simulink model "mpu6050"  (R2017b)
settings: Solver=FixedStepDiscrete  StartTime=0.0  StopTime=0.5  FixedStep=0.01  RelTol=1e-3
undefined symbols (not defined in the file): DiscIntNeverNeededParam, KiRollAttitude, KpRollAttitude, mpu6050
libraries: simulink x6, GPIO_Lib x3, TIMERS_Lib x2, STM32_Config_Lib x1
(part 1 of 2)
settings Model: Creator=edupc  LastModifiedBy=edupc
settings OptimizationCC: DefaultParameterBehavior=Inlined  PassReuseOutputArgsAs=Individual arguments
settings DebuggingCC: ParameterTunabilityLossMsg=error
settings HardwareCC: ProdBitPerPointer=32  ProdBitPerSizeT=32  ProdBitPerPtrDiffT=32  ProdLargestAtomicInteger=Integer  ProdWordSize=32  ProdHWDeviceType=STMicroelectronics->STM32 32-bit Cortex-M
settings SFSimCC: SimCustomHeaderCode="#include \"mac.h\""  SimUserSources=mac.c  MATLABDynamicMemAlloc=off
settings RTWCC: SystemTargetFile=stm32.tlc  TemplateMakefile=stm32.tmf  Description=stm32 (Embedded Target)  GenerateReport=on  IncludeHyperlinkInReport=on  GenerateTraceInfo=on  GenerateTraceReport=on  GenerateTraceReportSl=on  GenerateTraceReportSf=on  GenerateTraceReportEml=on
settings RTWCC: CustomHeaderCode=|
  | #include "printfFile.h"
  | #include "global.h"
settings CodeAppCC: ForceParamTrailComments=on  IgnoreCustomStorageClasses=off  MaxIdLength=64  OperatorAnnotations=on  SimulinkDataObjDesc=on  SFDataObjDesc=on  CustomSymbolStrType=$N$R$M  SimulinkBlockComments=off
settings STFCustomTargetCC: CodeReplacementLibrary=ARM CMSIS SIN COS  MultiwordLength=256  ParMdlRefBuildCompliant=on  IncludeMdlTerminateFcn=off  CombineOutputUpdateFcns=on  ERTCustomFileBanners=on  SupportContinuousTime=off  SupportNonInlinedSFcns=off  RemoveResetFunc=on  MATLABClassNameForMDSCustomization=Simulink.SoftwareTarget.ERTCustomization  GRTInterface=off  SystemTargetFile=stm32.tlc
settings ERTTargetCC: CodeReplacementLibrary=ARM CMSIS SIN COS  CompOptLevelCompliant=off  ConcurrentExecutionCompliant=off  IncludeMdlTerminateFcn=off  ModelStepFunctionPrototypeControlCompliant=off  CPPClassGenCompliant=off  UseToolchainInfoCompliant=off  ExtModeStaticAllocSize=256  ExtModeMexArgs=0,1,115200,10  InlinedParameterPlacement=NonHierarchical  ERTSrcFileBannerTemplate=sourceFileTemplate.cgt  ERTHdrFileBannerTemplate=sourceFileTemplate.cgt  ERTDataSrcFileTemplate=sourceFileTemplate.cgt  ERTDataHdrFileTemplate=sourceFileTemplate.cgt  ERTCustomFileTemplate=customRoutineProcess.tlc

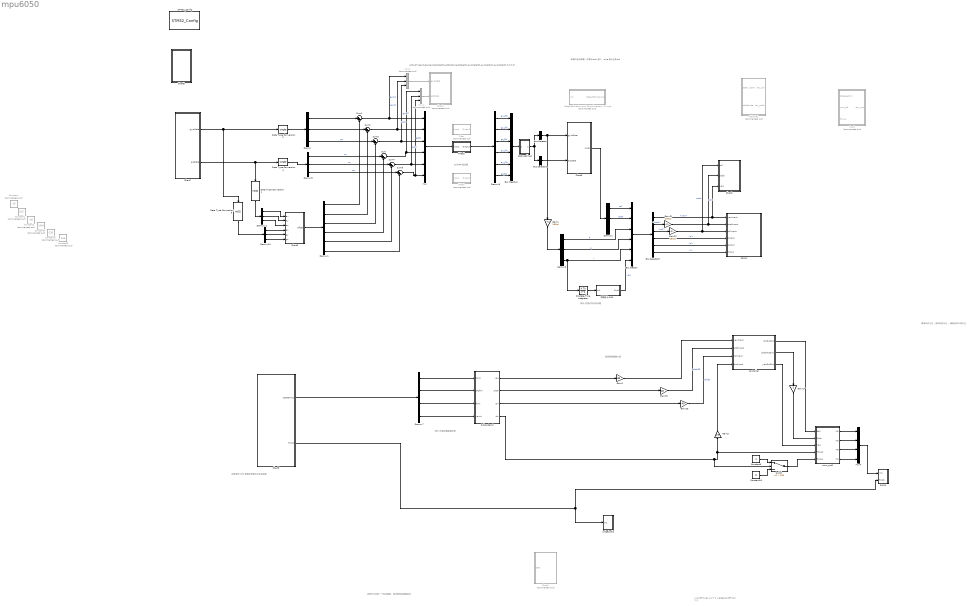
== system mpu6050 ==
  note: //				printf("over run");
      | 			}
      | //      else{printf("no\r\n");}
  note: 50Hz的遥控器数据处理
  note: 角速度期望最大值
  note: 10阶FIR滤波器
  note: ANO_DT_Send_Senser(accData[0],accData[1],accData[2],gyroData[0],gyroData[1],gyroData[2],0,0,0,0);
  note: 这里可以先放一个发送函数，测试是否有数据丢失
  note: 这里添加了PID参数回传确认的发送函数
  note: 航向 这里还存在些问题
  note: 横滚向右为正，俯仰向前为正，
      | 偏航逆时针转为正
  note: 移植的姿态解算，陀螺仪rad/s输入，ouler输出也是rad
  Attitude1 : Subsystem  Commented=on  TreatAsAtomicUnit=on
  Bus Creator : BusCreator  Inputs=6
  Bus Creator4 : BusCreator  Inputs=6
  Bus Selector : BusSelector  OutputSignals=p,q,r  OutputAsBus=on
  Bus Selector1 : BusSelector  OutputSignals=x_acc,y_acc,z_acc  OutputAsBus=on
  Bus Selector3 : BusSelector  OutputSignals=yaw,pitch,roll,p,q,r
  Chart1 : Stateflow chart  TreatAsAtomicUnit=on
  Chart2 : Stateflow chart  Commented=on  TreatAsAtomicUnit=on
  Chart3 : Stateflow chart  TreatAsAtomicUnit=on
  Chart4 : Stateflow chart  Commented=on  TreatAsAtomicUnit=on
  Chart5 : Stateflow chart  TreatAsAtomicUnit=on
  Chart6 : Stateflow chart  TreatAsAtomicUnit=on
  Chart7 : Stateflow chart  TreatAsAtomicUnit=on
  Chart8 : Stateflow chart  Priority=1  TreatAsAtomicUnit=on
  Constant : Constant  Commented=on  Value=-29  OutDataTypeStr=single
  Constant1 : Constant  Commented=on  Value=16.5  OutDataTypeStr=single
  Constant10 : Constant  Value=0  OutDataTypeStr=single
  Constant2 : Constant  Commented=on  Value=-36  OutDataTypeStr=single
  Constant3 : Constant  Commented=on  Value=1040  OutDataTypeStr=single
  Constant4 : Constant  Commented=on  Value=-130  OutDataTypeStr=single
  Constant5 : Constant  Commented=on  Value=516  OutDataTypeStr=single
  Constant9 : Constant  OutDataTypeStr=single
  Data Type Conversion1 : DataTypeConversion  OutDataTypeStr=int32
  Data Type Conversion2 : DataTypeConversion  OutDataTypeStr=single  RndMeth=Nearest
  Data Type Conversion4 : DataTypeConversion  OutDataTypeStr=single  RndMeth=Nearest
  Data Type Conversion5 : DataTypeConversion  OutDataTypeStr=int32
  Demux{,2..3,9..11} (6 alike) : Demux  Outputs=3
  Demux1 : Demux  Outputs=6
  Demux7 : Demux
  Demux8 : Demux  Outputs=6
  Discrete-Time Integrator : DiscreteIntegrator  gainval=1  InitialConditionSetting=State (most efficient)  SampleTime=-1  ICPrevOutput=DiscIntNeverNeededParam  ICPrevScaledInput=DiscIntNeverNeededParam
  Filter : Subsystem  Tag=FilterWizardSubSystem  Commented=on
      settings: ErrorFcn=dspFilterRealizedInBasicElemsAlgLoopErrFcnCallback
  Filter1 : Subsystem  Tag=FilterWizardSubSystem  Commented=on
      settings: ErrorFcn=dspFilterRealizedInBasicElemsAlgLoopErrFcnCallback
  Filter2 : Subsystem  Tag=FilterWizardSubSystem
      settings: ErrorFcn=dspFilterRealizedInBasicElemsAlgLoopErrFcnCallback
  Gain1 : Gain  Gain=180/pi
  Gain17 : Gain  Gain=-1  ParamDataTypeStr=single  OutDataTypeStr=single
  Gain19 : Gain  Gain=40  ParamDataTypeStr=single
  Gain2 : Gain  Gain=180  ParamDataTypeStr=single
  Gain20 : Gain  Gain=40
  Gain21 : Gain  Gain=180/pi
  Gain22 : Gain  Gain=180/pi
  Gain3 : Gain  Gain=0.5  ParamDataTypeStr=single
  Mux : Mux  Inputs=6
  Mux1 : Mux  Commented=on  Inputs=3
  Mux2 : Mux  Commented=on  Inputs=3
  Mux4 : Mux
  PWM1 : Subsystem  TreatAsAtomicUnit=on
  STM32_Config : STM32_Config_Lib/STM32_Config  Priority=0  Project_Path=.\mpu6050\  Config_File=mpu6050.ioc  MCU_Name=STM32F103T8Ux
      settings: SourceProductName=Target Support Package - STM32 Adapter
  State Estimation and Complimentary Mixing1 : Subsystem  Commented=on  mask{EAComp=0.95}
      mask prompts: EAComp "Complimentary Filter Alpha:"
      mask TypeOptions EAComp: Complimentary Filter/EAComp
  Subsystem2 : Subsystem  TreatAsAtomicUnit=on
  Sum{,1..5} (6 alike) : Sum  Inputs=|+-
  Switch : Switch  Criteria=u2 > Threshold  Threshold=100
  Yaw1 : Subsystem  Commented=on  TreatAsAtomicUnit=on
  controller : Stateflow chart  TreatAsAtomicUnit=on
  data scaling1 : Subsystem
  judgeLock2 : Subsystem  TreatAsAtomicUnit=on
  pwm_out2 : MATLAB Function  TreatAsAtomicUnit=on
  sensor : Stateflow chart  TreatAsAtomicUnit=on
  限幅到+-180， : Subsystem
  wires:
  Data Type Conversion1/1 -> Demux11/1
  Demux10/1 -> Chart6/4(gx)
  Demux1/6 -> Sum5/2
  Demux11/1 -> Chart6/1(ax)
  Demux1/4 -> Sum/2
  Demux10/2 -> Chart6/5(gy)
  Chart7/2(accData) -> Data Type Conversion1/1, Data Type Conversion4/1
  Sum/1 -> Mux1/1, Mux/4  "accX"
  Demux1/2 -> Sum2/2
  Demux/2 -> Sum2/1
  Data Type Conversion2/1 -> Demux/1
  Sum1/1 -> Mux2/1, Mux/1  "gyroX"
  Sum4/1 -> Mux1/2, Mux/5  "accY"
  Demux9/3 -> Sum5/1  "az"
  Demux11/2 -> Chart6/2(ay)
  Demux9/2 -> Sum4/1  "ay"
  Demux11/3 -> Chart6/3(az)
  Sum5/1 -> Mux1/3, Mux/6  "accZ"
  Demux9/1 -> Sum/1  "ax"
  Demux10/3 -> Chart6/6(gz)
  Chart7/1(gyroData) -> Data Type Conversion2/1, Data Type Conversion5/1
  Demux1/1 -> Sum1/2
  Sum3/1 -> Mux2/3, Mux/3  "gyroZ"
  Demux/3 -> Sum3/1  "gz"
  Demux/1 -> Sum1/1
  Data Type Conversion5/1 -> Demux10/1
  Data Type Conversion4/1 -> Demux9/1
  Demux1/5 -> Sum4/2
  Demux1/3 -> Sum3/2
  Sum2/1 -> Mux2/2, Mux/2  "gryoY"
  Demux8/5 -> Bus Creator4/5  "ay_filt"
  Demux8/1 -> Bus Creator4/1  "gx_filt"
  Mux/1 -> Filter2/1(Input)
  Demux8/2 -> Bus Creator4/2  "gy_filt"
  Demux8/3 -> Bus Creator4/3  "gz_filt"
  Demux8/4 -> Bus Creator4/4  "ax_filt"
  Bus Creator4/1 -> data scaling1/1(In1)
  Demux8/6 -> Bus Creator4/6  "az_filt"
  Chart5/1(rcDataTmp) -> Demux7/1
  controller/2(pitchOutSim) -> Gain17/1
  Mux4/1 -> PWM1/1(In1)
  Subsystem2/3(roll) -> Gain20/1
  pwm_out2/2(M2) -> Mux4/2
  Chart5/2(FlyOk) -> PWM1/2(flyOk), judgeLock2/1(In1)
  Demux7/4 -> Subsystem2/4(yawIn)
  Subsystem2/2(pitch) -> Gain19/1
  Subsystem2/1(yaw) -> Gain2/1
  pwm_out2/1(M1) -> Mux4/1
  pwm_out2/4(M4) -> Mux4/4
  pwm_out2/3(M3) -> Mux4/3
  Demux7/2 -> Subsystem2/2(pitchIn)
  Subsystem2/4(thr) -> Switch/2, pwm_out2/4(Thrust), Gain3/1
  Demux7/3 -> Subsystem2/3(thrIn)
  Demux7/1 -> Subsystem2/1(rollIn)
  Chart3/1(ouler) -> Demux2/1
  data scaling1/1(Out1) -> Bus Selector1/1, Bus Selector/1
  Bus Selector1/1 -> Chart3/2(accData)
  Bus Selector/1 -> Chart3/1(gyroData), Gain1/1
  Demux2/1 -> Bus Creator/1  "roll"
  Demux2/2 -> Bus Creator/2  "pitch"
  Bus Creator/1 -> Bus Selector3/1
  Demux3/1 -> Bus Creator/3  "p"
  Demux3/2 -> Bus Creator/4  "q"
  Demux3/3 -> Discrete-Time Integrator/1, Bus Creator/5  "r"
  Filter2/1(Output) -> Demux8/1
  Discrete-Time Integrator/1 -> 限幅到+-180，/1(In1)
  限幅到+-180，/1(Out1) -> Bus Creator/6  "yaw"
  Gain17/1 -> pwm_out2/2(Pitch)
  Chart6/1(offset) -> Demux1/1
  Mux1/1 -> Chart4/2(accData)
  Mux2/1 -> Chart4/1(gyroData)
  Gain2/1 -> controller/1(yawInput)
  Gain3/1 -> controller/4(throInput)
  Constant10/1 -> Switch/3
  Constant9/1 -> Switch/1
  Switch/1 -> pwm_out2/5(thrLow)
  Gain19/1 -> controller/2(pitchInput)  "pitchCtl"
  Gain20/1 -> controller/3(rollInput)  "rollCtl"
  Bus Selector3/1 -> Chart1/3(yaw), sensor/1(yawInput)  "<yaw>"
  Bus Selector3/2 -> Gain21/1  "<pitch>"
  Bus Selector3/3 -> Gain22/1  "<roll>"
  Gain21/1 -> Chart1/2(pitch), sensor/2(pitchInput)  "roll"
  Gain22/1 -> Chart1/1(roll), sensor/3(rollInput)  "pitch"
  Bus Selector3/4 -> sensor/4(pInput)  "<p>"
  Bus Selector3/5 -> sensor/5(qInput)  "<q>"
  Bus Selector3/6 -> sensor/6(rInput)  "<r>"
  controller/3(yawOutSim) -> pwm_out2/3(Yaw)
  Gain1/1 -> Demux3/1
  controller/1(rollOutSim) -> pwm_out2/1(Roll)

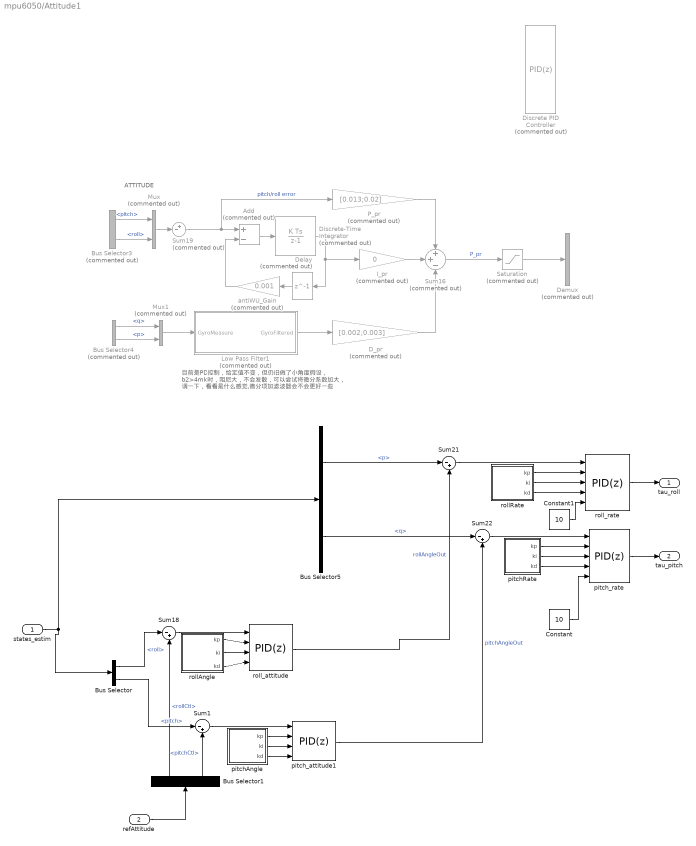
== system mpu6050/Attitude1 ==
  note: 目前是PD控制，给定值不变，但仍旧做了小角度假设，
      | b2>4mk时，阻尼大，不会发散，可以尝试将微分系数加大，
      | 调一下，看看是什么感觉,微分项加滤波器会不会更好一些
  note: ATTITUDE
  states_estim : Inport
  refAttitude : Inport  Port=2
  Add : Sum  Commented=on  Inputs=+-
  Bus Selector : BusSelector  OutputSignals=roll,pitch
  Bus Selector1 : BusSelector  OutputSignals=rollCtl,pitchCtl
  Bus Selector3 : BusSelector  Commented=on  OutputSignals=pitch,roll
  Bus Selector4 : BusSelector  Commented=on  OutputSignals=q,p
  Bus Selector5 : BusSelector  OutputSignals=p,q
  Constant : Constant  Value=10  OutDataTypeStr=int8
  Constant1 : Constant  Value=10  OutDataTypeStr=int8
  D_pr : Gain  Commented=on  Gain=[0.002;0.003]  ParamDataTypeStr=single  OutDataTypeStr=single
  Delay : Delay  Commented=on  DelayLength=1  InitialCondition=0
  Demux : Demux  Commented=on  Outputs=2
  Discrete PID Controller : simulink/Continuous/PID Controller  Commented=on  Controller=PID  TimeDomain=Discrete-time  SampleTime=-1  IntegratorMethod=Backward Euler  FilterMethod=Backward Euler  Form=Parallel  UseFilter=on  ControllerParametersSource=external  P=1  I=1  D=0  N=100  InitialConditionSource=internal  InitialConditionForIntegrator=0  InitialConditionForFilter=0  ExternalReset=none  LimitOutput=off  UpperSaturationLimit=inf  LowerSaturationLimit=-inf  LinearizeAsGain=off  AntiWindupMode=none  Kb=1  TrackingMode=off  Kt=1  PParamMin=[]  PParamMax=[]  IParamMin=[]  IParamMax=[]  DParamMin=[]  DParamMax=[]  NParamMin=[]  NParamMax=[]  KbParamMin=[]  KbParamMax=[]  KtParamMin=[]  KtParamMax=[]  POutMin=[]  POutMax=[]  IOutMin=[]  IOutMax=[]  DOutMin=[]  DOutMax=[]  NOutMin=[]  NOutMax=[]  KbOutMin=[]  KbOutMax=[]  KtOutMin=[]  KtOutMax=[]  IntegratorOutMin=[]  IntegratorOutMax=[]  FilterOutMin=[]  FilterOutMax=[]  SumOutMin=[]  SumOutMax=[]  SumI1OutMin=[]  SumI1OutMax=[]  SumI2OutMin=[]  SumI2OutMax=[]  SumI3OutMin=[]  SumI3OutMax=[]  SumDOutMin=[]  SumDOutMax=[]  SaturationOutMin=[]  SaturationOutMax=[]  IntegratorContinuousStateAttributes=''  IntegratorStateMustResolveToSignalObject=off  IntegratorRTWStateStorageClass=Auto  FilterContinuousStateAttributes=''  FilterStateMustResolveToSignalObject=off  FilterRTWStateStorageClass=Auto  DifferentiatorICPrevScaledInput=0  DifferentiatorOutMin=[]  DifferentiatorOutMax=[]  InitialConditionSetting=State (most efficient)  FilterDiffOutCoefMin=[]  FilterDiffOutCoefMax=[]  SumDenOutMin=[]  SumDenOutMax=[]  SumNumOutMin=[]  SumNumOutMax=[]  ReciprocalOutMin=[]  ReciprocalOutMax=[]  DivideOutMin=[]  DivideOutMax=[]  TunerSelectOption=Transfer Function Based (PID Tuner App)
  Discrete-Time Integrator : DiscreteIntegrator  Commented=on  InitialConditionSetting=State (most efficient)  SampleTime=-1  LimitOutput=on  UpperSaturationLimit=0.1  LowerSaturationLimit=-0.1  ICPrevOutput=DiscIntNeverNeededParam  ICPrevScaledInput=DiscIntNeverNeededParam
  I_pr : Gain  Commented=on  Gain=0  ParamDataTypeStr=single  OutDataTypeStr=single
  Low Pass Filter1 : Subsystem  Commented=on
  Mux : Mux  Commented=on  Inputs=2
  Mux1 : Mux  Commented=on  Inputs=2
  P_pr : Gain  Commented=on  Gain=[0.013;0.02]  ParamDataTypeStr=single  OutDataTypeStr=single
  Saturation : Saturate  Commented=on  UpperLimit=0.2  LowerLimit=-0.2
  Sum{1,18,21..22} (4 alike) : Sum  Inputs=|-+
  Sum16 : Sum  Commented=on  Inputs=++-  AccumDataTypeStr=single  OutDataTypeStr=single  SaturateOnIntegerOverflow=on
  Sum19 : Sum  Commented=on  Inputs=+-|
  antiWU_Gain : Gain  Commented=on  Gain=0.001
  pitchAngle : Stateflow chart  TreatAsAtomicUnit=on
  pitchRate : Stateflow chart  TreatAsAtomicUnit=on
  pitch_attitude1 : simulink/Continuous/PID Controller  Controller=PID  TimeDomain=Discrete-time  SampleTime=-1  IntegratorMethod=Forward Euler  FilterMethod=Forward Euler  Form=Parallel  UseFilter=off  ControllerParametersSource=external  P=KpRollAttitude  I=KiRollAttitude  D=0.01  N=100  InitialConditionSource=internal  InitialConditionForIntegrator=0  InitialConditionForFilter=0  ExternalReset=none  LimitOutput=on  UpperSaturationLimit=300  LowerSaturationLimit=-300  LinearizeAsGain=on  AntiWindupMode=back-calculation  Kb=2  TrackingMode=off  Kt=1  PParamMin=[]  PParamMax=[]  IParamMin=[]  IParamMax=[]  DParamMin=[]  DParamMax=[]  NParamMin=[]  NParamMax=[]  KbParamMin=[]  KbParamMax=[]  KtParamMin=[]  KtParamMax=[]  POutMin=[]  POutMax=[]  IOutMin=[-10]  IOutMax=[10]  DOutMin=[]  DOutMax=[]  NOutMin=[]  NOutMax=[]  KbOutMin=[]  KbOutMax=[]  KtOutMin=[]  KtOutMax=[]  IntegratorOutMin=[]  IntegratorOutMax=[]  FilterOutMin=[]  FilterOutMax=[]  SumOutMin=[]  SumOutMax=[]  SumI1OutMin=[]  SumI1OutMax=[]  SumI2OutMin=[]  SumI2OutMax=[]  SumI3OutMin=[]  SumI3OutMax=[]  SumDOutMin=[]  SumDOutMax=[]  SaturationOutMin=[]  SaturationOutMax=[]  IntegratorContinuousStateAttributes=''  IntegratorStateMustResolveToSignalObject=off  IntegratorRTWStateStorageClass=Auto  FilterContinuousStateAttributes=''  FilterStateMustResolveToSignalObject=off  FilterRTWStateStorageClass=Auto  DifferentiatorICPrevScaledInput=0  DifferentiatorOutMin=[]  DifferentiatorOutMax=[]  InitialConditionSetting=State (most efficient)  FilterDiffOutCoefMin=[]  FilterDiffOutCoefMax=[]  SumDenOutMin=[]  SumDenOutMax=[]  SumNumOutMin=[]  SumNumOutMax=[]  ReciprocalOutMin=[]  ReciprocalOutMax=[]  DivideOutMin=[]  DivideOutMax=[]  TunerSelectOption=Transfer Function Based (PID Tuner App)
  pitch_rate : simulink/Continuous/PID Controller  Controller=PID  TimeDomain=Discrete-time  SampleTime=-1  IntegratorMethod=Forward Euler  FilterMethod=Forward Euler  Form=Parallel  UseFilter=on  ControllerParametersSource=external  P=KpRollAttitude  I=KiRollAttitude  D=0.01  N=100  InitialConditionSource=internal  InitialConditionForIntegrator=0  InitialConditionForFilter=0  ExternalReset=none  LimitOutput=on  UpperSaturationLimit=300  LowerSaturationLimit=-300  LinearizeAsGain=on  AntiWindupMode=clamping  Kb=2  TrackingMode=off  Kt=1  PParamMin=[]  PParamMax=[]  IParamMin=[]  IParamMax=[]  DParamMin=[]  DParamMax=[]  NParamMin=[]  NParamMax=[]  KbParamMin=[]  KbParamMax=[]  KtParamMin=[]  KtParamMax=[]  POutMin=[]  POutMax=[]  IOutMin=[]  IOutMax=[]  DOutMin=[]  DOutMax=[]  NOutMin=[]  NOutMax=[]  KbOutMin=[]  KbOutMax=[]  KtOutMin=[]  KtOutMax=[]  IntegratorOutMin=[-100]  IntegratorOutMax=[100]  FilterOutMin=[]  FilterOutMax=[]  SumOutMin=[]  SumOutMax=[]  SumI1OutMin=[]  SumI1OutMax=[]  SumI2OutMin=[]  SumI2OutMax=[]  SumI3OutMin=[]  SumI3OutMax=[]  SumDOutMin=[]  SumDOutMax=[]  SaturationOutMin=[]  SaturationOutMax=[]  IntegratorContinuousStateAttributes=''  IntegratorStateMustResolveToSignalObject=off  IntegratorRTWStateStorageClass=Auto  FilterContinuousStateAttributes=''  FilterStateMustResolveToSignalObject=off  FilterRTWStateStorageClass=Auto  DifferentiatorICPrevScaledInput=0  DifferentiatorOutMin=[]  DifferentiatorOutMax=[]  InitialConditionSetting=State (most efficient)  FilterDiffOutCoefMin=[]  FilterDiffOutCoefMax=[]  SumDenOutMin=[]  SumDenOutMax=[]  SumNumOutMin=[]  SumNumOutMax=[]  ReciprocalOutMin=[]  ReciprocalOutMax=[]  DivideOutMin=[]  DivideOutMax=[]  TunerSelectOption=Transfer Function Based (PID Tuner App)
  rollAngle : Stateflow chart  TreatAsAtomicUnit=on
  rollRate : Stateflow chart  TreatAsAtomicUnit=on
  roll_attitude : simulink/Continuous/PID Controller  Controller=PID  TimeDomain=Discrete-time  SampleTime=-1  IntegratorMethod=Forward Euler  FilterMethod=Forward Euler  Form=Parallel  UseFilter=off  ControllerParametersSource=external  P=KpRollAttitude  I=KiRollAttitude  D=0.01  N=100  InitialConditionSource=internal  InitialConditionForIntegrator=0  InitialConditionForFilter=0  ExternalReset=none  LimitOutput=on  UpperSaturationLimit=300  LowerSaturationLimit=-300  LinearizeAsGain=on  AntiWindupMode=back-calculation  Kb=2  TrackingMode=off  Kt=1  PParamMin=[]  PParamMax=[]  IParamMin=[]  IParamMax=[]  DParamMin=[]  DParamMax=[]  NParamMin=[]  NParamMax=[]  KbParamMin=[]  KbParamMax=[]  KtParamMin=[]  KtParamMax=[]  POutMin=[]  POutMax=[]  IOutMin=[-10]  IOutMax=[10]  DOutMin=[]  DOutMax=[]  NOutMin=[]  NOutMax=[]  KbOutMin=[]  KbOutMax=[]  KtOutMin=[]  KtOutMax=[]  IntegratorOutMin=[]  IntegratorOutMax=[]  FilterOutMin=[]  FilterOutMax=[]  SumOutMin=[]  SumOutMax=[]  SumI1OutMin=[]  SumI1OutMax=[]  SumI2OutMin=[]  SumI2OutMax=[]  SumI3OutMin=[]  SumI3OutMax=[]  SumDOutMin=[]  SumDOutMax=[]  SaturationOutMin=[]  SaturationOutMax=[]  IntegratorContinuousStateAttributes=''  IntegratorStateMustResolveToSignalObject=off  IntegratorRTWStateStorageClass=Auto  FilterContinuousStateAttributes=''  FilterStateMustResolveToSignalObject=off  FilterRTWStateStorageClass=Auto  DifferentiatorICPrevScaledInput=0  DifferentiatorOutMin=[]  DifferentiatorOutMax=[]  InitialConditionSetting=State (most efficient)  FilterDiffOutCoefMin=[]  FilterDiffOutCoefMax=[]  SumDenOutMin=[]  SumDenOutMax=[]  SumNumOutMin=[]  SumNumOutMax=[]  ReciprocalOutMin=[]  ReciprocalOutMax=[]  DivideOutMin=[]  DivideOutMax=[]  TunerSelectOption=Transfer Function Based (PID Tuner App)
  roll_rate : simulink/Continuous/PID Controller  Controller=PID  TimeDomain=Discrete-time  SampleTime=-1  IntegratorMethod=Forward Euler  FilterMethod=Forward Euler  Form=Parallel  UseFilter=on  ControllerParametersSource=external  P=KpRollAttitude  I=KiRollAttitude  D=0.01  N=100  InitialConditionSource=internal  InitialConditionForIntegrator=0  InitialConditionForFilter=0  ExternalReset=none  LimitOutput=on  UpperSaturationLimit=300  LowerSaturationLimit=-300  LinearizeAsGain=on  AntiWindupMode=clamping  Kb=2  TrackingMode=off  Kt=1  PParamMin=[]  PParamMax=[]  IParamMin=[]  IParamMax=[]  DParamMin=[]  DParamMax=[]  NParamMin=[]  NParamMax=[]  KbParamMin=[]  KbParamMax=[]  KtParamMin=[]  KtParamMax=[]  POutMin=[]  POutMax=[]  IOutMin=[]  IOutMax=[]  DOutMin=[]  DOutMax=[]  NOutMin=[]  NOutMax=[]  KbOutMin=[]  KbOutMax=[]  KtOutMin=[]  KtOutMax=[]  IntegratorOutMin=[-100]  IntegratorOutMax=[100]  FilterOutMin=[]  FilterOutMax=[]  SumOutMin=[]  SumOutMax=[]  SumI1OutMin=[]  SumI1OutMax=[]  SumI2OutMin=[]  SumI2OutMax=[]  SumI3OutMin=[]  SumI3OutMax=[]  SumDOutMin=[]  SumDOutMax=[]  SaturationOutMin=[]  SaturationOutMax=[]  IntegratorContinuousStateAttributes=''  IntegratorStateMustResolveToSignalObject=off  IntegratorRTWStateStorageClass=Auto  FilterContinuousStateAttributes=''  FilterStateMustResolveToSignalObject=off  FilterRTWStateStorageClass=Auto  DifferentiatorICPrevScaledInput=0  DifferentiatorOutMin=[]  DifferentiatorOutMax=[]  InitialConditionSetting=State (most efficient)  FilterDiffOutCoefMin=[]  FilterDiffOutCoefMax=[]  SumDenOutMin=[]  SumDenOutMax=[]  SumNumOutMin=[]  SumNumOutMax=[]  ReciprocalOutMin=[]  ReciprocalOutMax=[]  DivideOutMin=[]  DivideOutMax=[]  TunerSelectOption=Transfer Function Based (PID Tuner App)
  tau_roll : Outport
  tau_pitch : Outport  Port=2
  wires:
  Mux1/1 -> Low Pass Filter1/1(GyroMeasure)
  Bus Selector4/2 -> Mux1/2  "<p>"
  Bus Selector3/2 -> Mux/2  "<roll>"
  Mux/1 -> Sum19/2
  D_pr/1 -> Sum16/3
  Delay/1 -> antiWU_Gain/1
  Discrete-Time Integrator/1 -> I_pr/1, Delay/1
  Sum19/1 -> P_pr/1, Add/1  "pitch/roll error"
  I_pr/1 -> Sum16/2
  P_pr/1 -> Sum16/1
  Bus Selector4/1 -> Mux1/1  "<q>"
  Bus Selector3/1 -> Mux/1  "<pitch>"
  Add/1 -> Discrete-Time Integrator/1
  antiWU_Gain/1 -> Add/2
  Sum16/1 -> Saturation/1  "P_pr"
  Saturation/1 -> Demux/1
  Low Pass Filter1/1(GyroFiltered) -> D_pr/1
  Sum18/1 -> roll_attitude/1
  Sum21/1 -> roll_rate/1
  Sum1/1 -> pitch_attitude1/1
  roll_rate/1 -> tau_roll/1
  Bus Selector5/1 -> Sum21/1  "<p>"
  pitch_rate/1 -> tau_pitch/1
  roll_attitude/1 -> Sum21/2  "rollAngleOut"
  Bus Selector1/2 -> Sum1/2  "<pitchCtl>"
  pitch_attitude1/1 -> Sum22/2  "pitchAngleOut"
  Bus Selector1/1 -> Sum18/2  "<rollCtl>"
  Sum22/1 -> pitch_rate/1
  Bus Selector/2 -> Sum1/1  "<pitch>"
  Bus Selector/1 -> Sum18/1  "<roll>"
  Bus Selector5/2 -> Sum22/1  "<q>"
  rollAngle/1(kp) -> roll_attitude/2
  rollAngle/2(ki) -> roll_attitude/3
  rollAngle/3(kd) -> roll_attitude/4
  pitchAngle/2(ki) -> pitch_attitude1/3
  pitchAngle/1(kp) -> pitch_attitude1/2
  pitchAngle/3(kd) -> pitch_attitude1/4
  pitchRate/1(kp) -> pitch_rate/2
  pitchRate/2(ki) -> pitch_rate/3
  pitchRate/3(kd) -> pitch_rate/4
  rollRate/1(kp) -> roll_rate/2
  rollRate/2(ki) -> roll_rate/3
  rollRate/3(kd) -> roll_rate/4
  Constant/1 -> pitch_rate/5
  Constant1/1 -> roll_rate/5
  refAttitude/1 -> Bus Selector1/1
  states_estim/1 -> Bus Selector5/1, Bus Selector/1

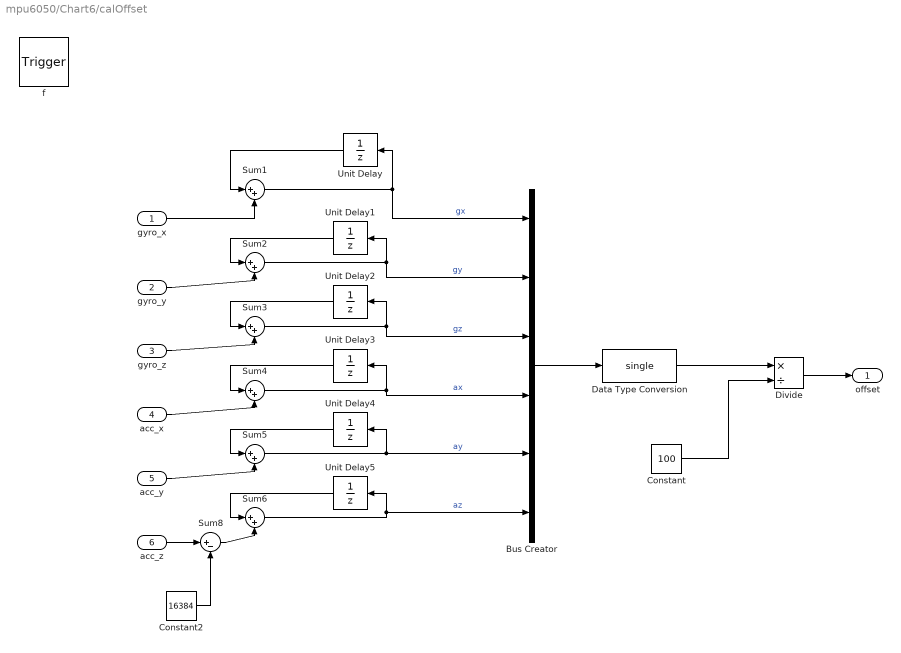
== system mpu6050/Chart6/calOffset ==
  gyro_x : Inport  OutDataTypeStr=int32
  gyro_y : Inport  Port=2  OutDataTypeStr=int32
  gyro_z : Inport  Port=3  OutDataTypeStr=int32
  acc_x : Inport  Port=4  OutDataTypeStr=int32
  acc_y : Inport  Port=5  OutDataTypeStr=int32
  acc_z : Inport  Port=6  OutDataTypeStr=int32
  f : TriggerPort  TriggerType=function-call  VariantControl=(inherit)
      settings: CopyFcn=Stateflow.SLINSF.SimulinkMan.removeBlockPreDeleteFcn  PreDeleteFcn=Stateflow.SLINSF.SimulinkMan.unsafePredeleteFcn
  Bus Creator : BusCreator  Inputs=6
  Constant : Constant  Value=100  OutDataTypeStr=single
  Constant2 : Constant  Value=16384  OutDataTypeStr=int16  SampleTime=-1
  Data Type Conversion : DataTypeConversion  OutDataTypeStr=single
  Divide : Product  Inputs=*/  OutDataTypeStr=single
  Sum{1..6} (6 alike) : Sum  Inputs=|++
  Sum8 : Sum  Inputs=|+-
  Unit Delay{,1..5} (6 alike) : UnitDelay  SampleTime=-1
  offset : Outport  OutDataTypeStr=single
  wires:
  gyro_x/1 -> Sum1/2
  Sum1/1 -> Bus Creator/1, Unit Delay/1  "gx"
  Unit Delay/1 -> Sum1/1
  gyro_y/1 -> Sum2/2
  Sum2/1 -> Unit Delay1/1, Bus Creator/2  "gy"
  Unit Delay1/1 -> Sum2/1
  Unit Delay2/1 -> Sum3/1
  Sum3/1 -> Unit Delay2/1, Bus Creator/3  "gz"
  Sum4/1 -> Unit Delay3/1, Bus Creator/4  "ax"
  Unit Delay3/1 -> Sum4/1
  Unit Delay4/1 -> Sum5/1
  Sum5/1 -> Unit Delay4/1, Bus Creator/5  "ay"
  Sum6/1 -> Bus Creator/6, Unit Delay5/1  "az"
  Unit Delay5/1 -> Sum6/1
  gyro_z/1 -> Sum3/2
  acc_x/1 -> Sum4/2
  acc_y/1 -> Sum5/2
  Bus Creator/1 -> Data Type Conversion/1
  acc_z/1 -> Sum8/1
  Sum8/1 -> Sum6/2
  Constant2/1 -> Sum8/2
  Constant/1 -> Divide/2
  Data Type Conversion/1 -> Divide/1
  Divide/1 -> offset/1

== system mpu6050/Chart8/BTInit ==
  f : TriggerPort  TriggerType=function-call  VariantControl=(inherit)
      settings: CopyFcn=Stateflow.SLINSF.SimulinkMan.removeBlockPreDeleteFcn  PreDeleteFcn=Stateflow.SLINSF.SimulinkMan.unsafePredeleteFcn
  Constant : Constant  OutDataTypeStr=int8
  GPIO_Write : GPIO_Lib/GPIO_Write  Port_name=GPIOB  Pin0=off  Toggle_Pin0=off  Pin1=off  Toggle_Pin1=off  Pin2=on  Toggle_Pin2=off  Pin3=off  Toggle_Pin3=off  Pin4=off  Toggle_Pin4=off  Pin5=off  Toggle_Pin5=off  Pin6=off  Toggle_Pin6=off  Pin7=off  Toggle_Pin7=off  Pin8=off  Toggle_Pin8=off  Pin9=off  Toggle_Pin9=off  Pin10=off  Toggle_Pin10=off  Pin11=off  Toggle_Pin11=off  Pin12=off  Toggle_Pin12=off  Pin13=off  Toggle_Pin13=off  Pin14=off  Toggle_Pin14=off  Pin15=off  Toggle_Pin15=off  PinList="GPIOA4   8  11  12GPIOB1  2  3  6  7"
      settings: SourceProductName=Target Support Package - STM32 Adapter
  wires:
  Constant/1 -> GPIO_Write/1

== system mpu6050/Chart8/pwmInit ==
  note: 模块内部初始值最好不要和设置的一样,同样要设置的小一些，
      | 比如25，这样占空比是1%
  f : TriggerPort  TriggerType=function-call  VariantControl=(inherit)
      settings: CopyFcn=Stateflow.SLINSF.SimulinkMan.removeBlockPreDeleteFcn  PreDeleteFcn=Stateflow.SLINSF.SimulinkMan.unsafePredeleteFcn
  Constant{1..4} (4 alike) : Constant  Value=0  OutDataTypeStr=int8
  Timers : TIMERS_Lib/Timers  Priority=1  currentTIM=TIM2  TIM_Name=TIM2  TIM_APBClock=72000000  TIM_Set_Clk=on  TIM_Prescaler=71  TIM_Clock=1000000.00  Variable_frequency=off  TIM_Set_OutFreq=on  TIM_ARR=2500  Output_frequency=400.00  Repetition_counter=0  TIM_Mode=Up  TIM_DMA=none  TIM_IRQ=off  TIM_IRQ_ONLY=off  TIM_UP=off  TIM_TRG=off  TIM_COM=off  TIM_BRK=off  NbTIM=2  CH1_enable=on  CH1N_enable=off  CH1_type=Output_PWM  CH1_DMA=off  CH1_int=off  CH1_edge=Rising  CH1_div=1  CH1_variable_duty=on  CH1_set_pulse=off  CH1_output_duty=1.00  CH1_pulse=25  CH2_enable=on  CH2N_enable=off  CH2_type=Output_PWM  CH2_DMA=off  CH2_int=off  CH2_edge=Rising  CH2_div=1  CH2_variable_duty=on  CH2_set_pulse=off  CH2_output_duty=1.00  CH2_pulse=25  CH3_enable=on  CH3N_enable=off  CH3_type=Output_PWM  CH3_DMA=off  CH3_int=off  CH3_edge=Rising  CH3_div=1  CH3_variable_duty=on  CH3_set_pulse=off  CH3_output_duty=1.00  CH3_pulse=25  CH4_enable=on  CH4N_enable=off  CH4_type=Output_PWM  CH4_DMA=off  CH4_int=off  CH4_edge=Rising  CH4_div=1  CH4_variable_duty=on  CH4_set_pulse=off  CH4_output_duty=1.00  CH4_pulse=25
      settings: SourceProductName=Target Support Package - STM32 Adapter
  wires:
  Constant2/1 -> Timers/2
  Constant1/1 -> Timers/1
  Constant3/1 -> Timers/3
  Constant4/1 -> Timers/4

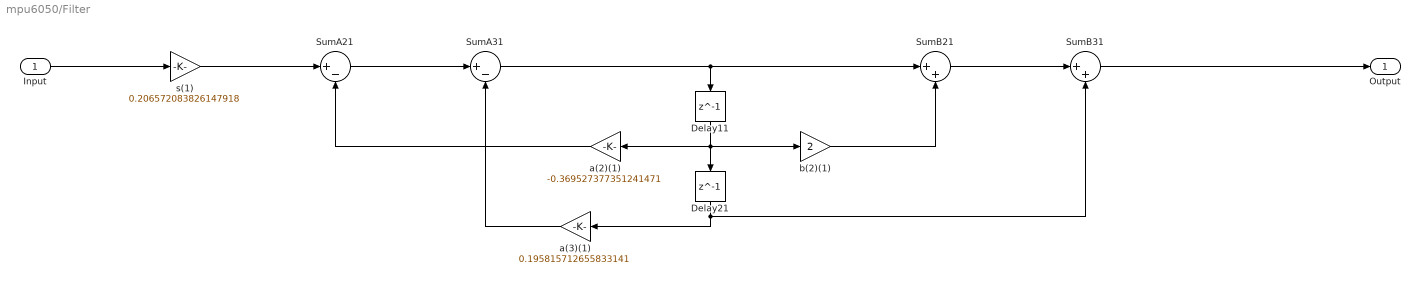
== system mpu6050/Filter ==
  Input : Inport
  Delay11 : Delay  DelayLength=1  InitialCondition=0
  Delay21 : Delay  DelayLength=1  InitialCondition=0
  SumA21 : Sum  Inputs=|+-  RndMeth=Nearest  SaturateOnIntegerOverflow=on  OutDataTypeStr=Inherit: Same as first input
  SumA31 : Sum  Inputs=|+-  RndMeth=Nearest  SaturateOnIntegerOverflow=on  OutDataTypeStr=Inherit: Same as first input
  SumB21 : Sum  Inputs=|++  RndMeth=Nearest  SaturateOnIntegerOverflow=on  OutDataTypeStr=Inherit: Same as first input
  SumB31 : Sum  Inputs=|++  RndMeth=Nearest  SaturateOnIntegerOverflow=on  OutDataTypeStr=Inherit: Same as first input
  a(2)(1) : Gain  Gain=-0.369527377351241471  ParamDataTypeStr=single  RndMeth=Nearest  SaturateOnIntegerOverflow=on  OutDataTypeStr=Inherit: Same as input
  a(3)(1) : Gain  Gain=0.195815712655833141  ParamDataTypeStr=single  RndMeth=Nearest  SaturateOnIntegerOverflow=on  OutDataTypeStr=Inherit: Same as input
  b(2)(1) : Gain  Gain=2  ParamDataTypeStr=single  RndMeth=Nearest  SaturateOnIntegerOverflow=on  OutDataTypeStr=Inherit: Same as input
  s(1) : Gain  Gain=0.206572083826147918  ParamDataTypeStr=single  RndMeth=Nearest  SaturateOnIntegerOverflow=on  OutDataTypeStr=Inherit: Same as input
  Output : Outport
  wires:
  Input/1 -> s(1)/1
  s(1)/1 -> SumA21/1
  SumA21/1 -> SumA31/1
  SumA31/1 -> SumB21/1, Delay11/1
  SumB21/1 -> SumB31/1
  SumB31/1 -> Output/1
  a(2)(1)/1 -> SumA21/2
  Delay11/1 -> a(2)(1)/1, b(2)(1)/1, Delay21/1
  b(2)(1)/1 -> SumB21/2
  a(3)(1)/1 -> SumA31/2
  Delay21/1 -> a(3)(1)/1, SumB31/2

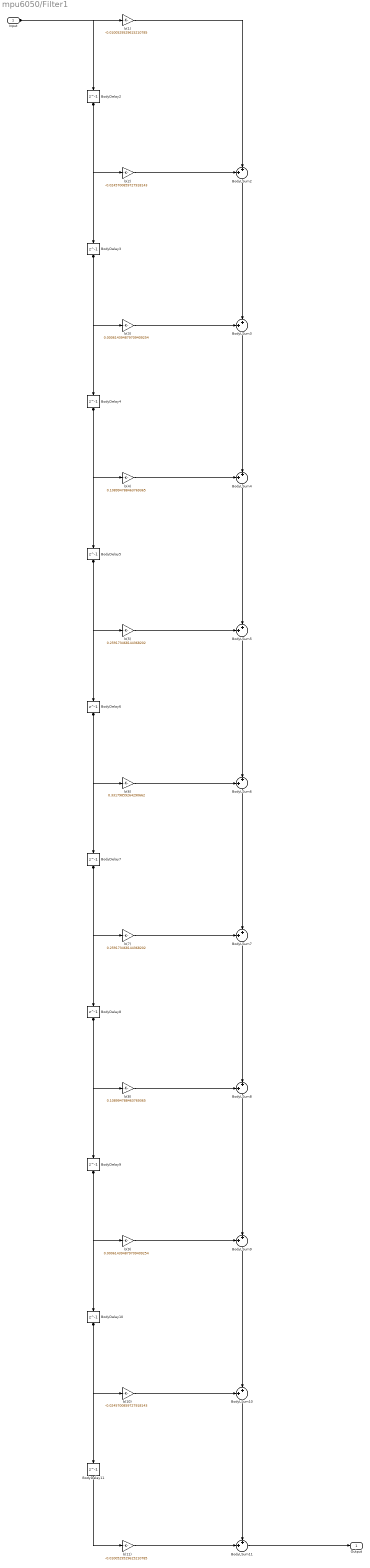
== system mpu6050/Filter1 ==
  Input : Inport
  BodyDelay{2..11} (10 alike) : Delay  DelayLength=1  InitialCondition=0  InputProcessing=Columns as channels (frame based)
  BodyLSum{2..11} (10 alike) : Sum  Inputs=++|  RndMeth=Nearest  SaturateOnIntegerOverflow=on  OutDataTypeStr=Inherit: Same as first input
  b(1) : Gain  Gain=-0.0100529529615210785  ParamDataTypeStr=single  RndMeth=Nearest  SaturateOnIntegerOverflow=on  OutDataTypeStr=Inherit: Same as input
  b(10) : Gain  Gain=-0.0245700859727918143  ParamDataTypeStr=single  RndMeth=Nearest  SaturateOnIntegerOverflow=on  OutDataTypeStr=Inherit: Same as input
  b(11) : Gain  Gain=-0.0100529529615210785  ParamDataTypeStr=single  RndMeth=Nearest  SaturateOnIntegerOverflow=on  OutDataTypeStr=Inherit: Same as input
  b(2) : Gain  Gain=-0.0245700859727918143  ParamDataTypeStr=single  RndMeth=Nearest  SaturateOnIntegerOverflow=on  OutDataTypeStr=Inherit: Same as input
  b(3) : Gain  Gain=0.000614394879709409254  ParamDataTypeStr=single  RndMeth=Nearest  SaturateOnIntegerOverflow=on  OutDataTypeStr=Inherit: Same as input
  b(4) : Gain  Gain=0.108994788463769365  ParamDataTypeStr=single  RndMeth=Nearest  SaturateOnIntegerOverflow=on  OutDataTypeStr=Inherit: Same as input
  b(5) : Gain  Gain=0.259173468144368202  ParamDataTypeStr=single  RndMeth=Nearest  SaturateOnIntegerOverflow=on  OutDataTypeStr=Inherit: Same as input
  b(6) : Gain  Gain=0.33179859264290662  ParamDataTypeStr=single  RndMeth=Nearest  SaturateOnIntegerOverflow=on  OutDataTypeStr=Inherit: Same as input
  b(7) : Gain  Gain=0.259173468144368202  ParamDataTypeStr=single  RndMeth=Nearest  SaturateOnIntegerOverflow=on  OutDataTypeStr=Inherit: Same as input
  b(8) : Gain  Gain=0.108994788463769365  ParamDataTypeStr=single  RndMeth=Nearest  SaturateOnIntegerOverflow=on  OutDataTypeStr=Inherit: Same as input
  b(9) : Gain  Gain=0.000614394879709409254  ParamDataTypeStr=single  RndMeth=Nearest  SaturateOnIntegerOverflow=on  OutDataTypeStr=Inherit: Same as input
  Output : Outport
  wires:
  Input/1 -> b(1)/1, BodyDelay2/1
  b(1)/1 -> BodyLSum2/2
  BodyDelay2/1 -> b(2)/1, BodyDelay3/1
  b(2)/1 -> BodyLSum2/1
  BodyLSum2/1 -> BodyLSum3/2
  BodyDelay3/1 -> b(3)/1, BodyDelay4/1
  b(3)/1 -> BodyLSum3/1
  BodyLSum3/1 -> BodyLSum4/2
  BodyDelay4/1 -> b(4)/1, BodyDelay5/1
  b(4)/1 -> BodyLSum4/1
  BodyLSum4/1 -> BodyLSum5/2
  BodyDelay5/1 -> b(5)/1, BodyDelay6/1
  b(5)/1 -> BodyLSum5/1
  BodyLSum5/1 -> BodyLSum6/2
  BodyDelay6/1 -> b(6)/1, BodyDelay7/1
  b(6)/1 -> BodyLSum6/1
  BodyLSum6/1 -> BodyLSum7/2
  BodyDelay7/1 -> b(7)/1, BodyDelay8/1
  b(7)/1 -> BodyLSum7/1
  BodyLSum7/1 -> BodyLSum8/2
  BodyDelay8/1 -> b(8)/1, BodyDelay9/1
  b(8)/1 -> BodyLSum8/1
  BodyLSum8/1 -> BodyLSum9/2
  BodyDelay9/1 -> b(9)/1, BodyDelay10/1
  b(9)/1 -> BodyLSum9/1
  BodyLSum9/1 -> BodyLSum10/2
  BodyDelay10/1 -> b(10)/1, BodyDelay11/1
  b(10)/1 -> BodyLSum10/1
  BodyLSum10/1 -> BodyLSum11/1
  BodyDelay11/1 -> b(11)/1
  b(11)/1 -> BodyLSum11/2
  BodyLSum11/1 -> Output/1

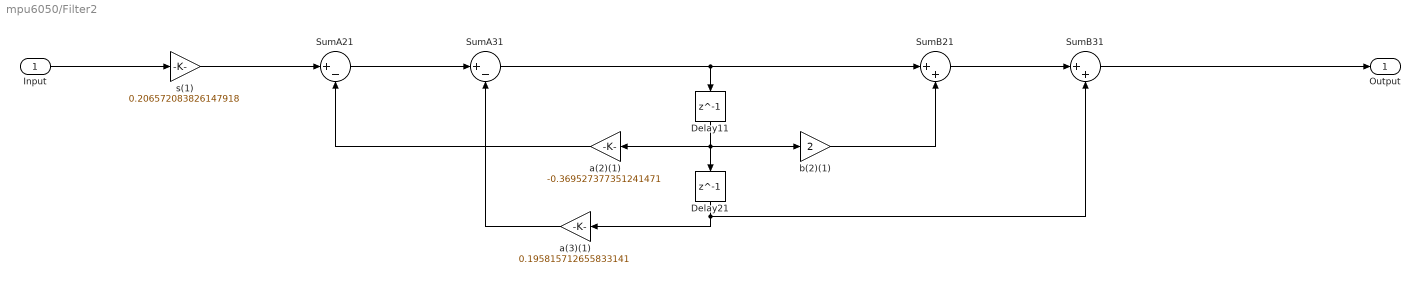
== system mpu6050/Filter2 ==
  Input : Inport
  Delay11 : Delay  DelayLength=1  InitialCondition=0
  Delay21 : Delay  DelayLength=1  InitialCondition=0
  SumA21 : Sum  Inputs=|+-  RndMeth=Nearest  SaturateOnIntegerOverflow=on  OutDataTypeStr=Inherit: Same as first input
  SumA31 : Sum  Inputs=|+-  RndMeth=Nearest  SaturateOnIntegerOverflow=on  OutDataTypeStr=Inherit: Same as first input
  SumB21 : Sum  Inputs=|++  RndMeth=Nearest  SaturateOnIntegerOverflow=on  OutDataTypeStr=Inherit: Same as first input
  SumB31 : Sum  Inputs=|++  RndMeth=Nearest  SaturateOnIntegerOverflow=on  OutDataTypeStr=Inherit: Same as first input
  a(2)(1) : Gain  Gain=-0.369527377351241471  ParamDataTypeStr=single  RndMeth=Nearest  SaturateOnIntegerOverflow=on  OutDataTypeStr=Inherit: Same as input
  a(3)(1) : Gain  Gain=0.195815712655833141  ParamDataTypeStr=single  RndMeth=Nearest  SaturateOnIntegerOverflow=on  OutDataTypeStr=Inherit: Same as input
  b(2)(1) : Gain  Gain=2  ParamDataTypeStr=single  RndMeth=Nearest  SaturateOnIntegerOverflow=on  OutDataTypeStr=Inherit: Same as input
  s(1) : Gain  Gain=0.206572083826147918  ParamDataTypeStr=single  RndMeth=Nearest  SaturateOnIntegerOverflow=on  OutDataTypeStr=Inherit: Same as input
  Output : Outport
  wires:
  Input/1 -> s(1)/1
  s(1)/1 -> SumA21/1
  SumA21/1 -> SumA31/1
  SumA31/1 -> SumB21/1, Delay11/1
  SumB21/1 -> SumB31/1
  SumB31/1 -> Output/1
  a(2)(1)/1 -> SumA21/2
  Delay11/1 -> a(2)(1)/1, b(2)(1)/1, Delay21/1
  b(2)(1)/1 -> SumB21/2
  a(3)(1)/1 -> SumA31/2
  Delay21/1 -> a(3)(1)/1, SumB31/2

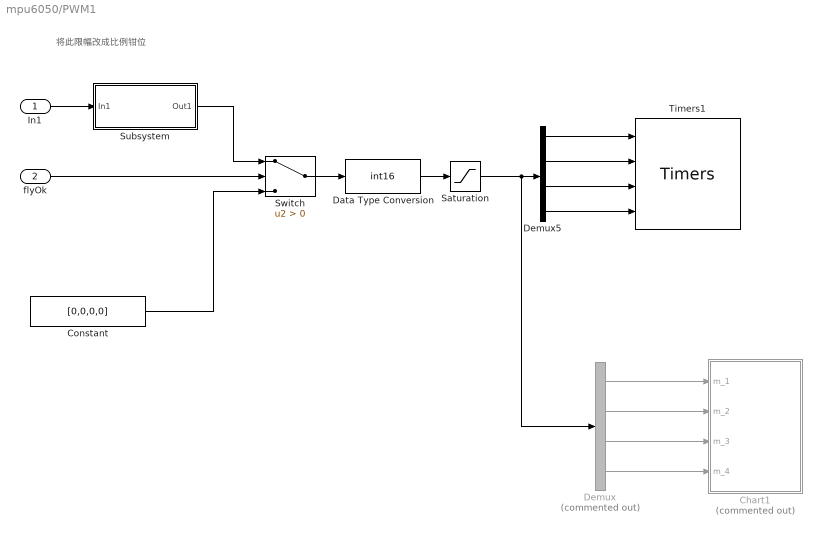
== system mpu6050/PWM1 ==
  note: 将此限幅改成比例钳位
  In1 : Inport
  flyOk : Inport  Port=2
  Chart1 : Stateflow chart  Commented=on  TreatAsAtomicUnit=on
  Constant : Constant  Value=[0,0,0,0]  OutDataTypeStr=single
  Data Type Conversion : DataTypeConversion  OutDataTypeStr=int16
  Demux : Demux  Commented=on
  Demux5 : Demux
  Saturation : Saturate  UpperLimit=1000  LowerLimit=0
  Subsystem : Subsystem
  Switch : Switch  Criteria=u2 > Threshold
  Timers1 : TIMERS_Lib/Timers  Priority=1  currentTIM=TIM2  TIM_Name=TIM2  TIM_APBClock=72000000  TIM_Set_Clk=on  TIM_Prescaler=71  TIM_Clock=1000000.00  Variable_frequency=off  TIM_Set_OutFreq=on  TIM_ARR=1000  Output_frequency=1000.00  Repetition_counter=0  TIM_Mode=Up  TIM_DMA=none  TIM_IRQ=off  TIM_IRQ_ONLY=off  TIM_UP=off  TIM_TRG=off  TIM_COM=off  TIM_BRK=off  NbTIM=2  CH1_enable=on  CH1N_enable=off  CH1_type=Output_PWM  CH1_DMA=off  CH1_int=off  CH1_edge=Rising  CH1_div=1  CH1_variable_duty=on  CH1_set_pulse=off  CH1_output_duty=1.00  CH1_pulse=10  CH2_enable=on  CH2N_enable=off  CH2_type=Output_PWM  CH2_DMA=off  CH2_int=off  CH2_edge=Rising  CH2_div=1  CH2_variable_duty=on  CH2_set_pulse=off  CH2_output_duty=1.00  CH2_pulse=10  CH3_enable=on  CH3N_enable=off  CH3_type=Output_PWM  CH3_DMA=off  CH3_int=off  CH3_edge=Rising  CH3_div=1  CH3_variable_duty=on  CH3_set_pulse=off  CH3_output_duty=1.00  CH3_pulse=10  CH4_enable=on  CH4N_enable=off  CH4_type=Output_PWM  CH4_DMA=off  CH4_int=off  CH4_edge=Rising  CH4_div=1  CH4_variable_duty=on  CH4_set_pulse=off  CH4_output_duty=1.00  CH4_pulse=10
      settings: SourceProductName=Target Support Package - STM32 Adapter
  wires:
  Switch/1 -> Data Type Conversion/1
  Demux5/1 -> Timers1/1
  Demux5/4 -> Timers1/4
  Demux5/2 -> Timers1/2
  Demux5/3 -> Timers1/3
  flyOk/1 -> Switch/2
  In1/1 -> Subsystem/1(In1)
  Data Type Conversion/1 -> Saturation/1
  Constant/1 -> Switch/3
  Subsystem/1(Out1) -> Switch/1
  Demux/1 -> Chart1/1(m_1)
  Demux/2 -> Chart1/2(m_2)
  Demux/3 -> Chart1/3(m_3)
  Demux/4 -> Chart1/4(m_4)
  Saturation/1 -> Demux/1, Demux5/1

== system mpu6050/State Estimation and Complimentary Mixing1 ==
  note: The specific state estimation procedure employed in these bocks is
      | to be considered experimental (like everything else in this simulation).
      | While functional within the context of our application, this is not to be taken
      | as a "correct" method for state estimation or gyro/accelerometer data combination.
  note: Note:
      | x_gyro is taken as P,
      | y_gyro as Q,
      | z_gyro ad R.
  In1 : Inport
  Bus Creator : BusCreator  Inputs=6
  Bus Selector : BusSelector  OutputSignals=p,q,r,x_acc,y_acc,z_acc
  Complimentary Filter : Subsystem  mask{EAComp=EAComp}
      mask prompts: EAComp "Complimentary Filter Alpha:"
      mask TypeOptions EAComp: EAComp1/Gain
  Subsystem1 : Subsystem
  State Estimations : Outport
  wires:
  In1/1 -> Bus Selector/1
  Bus Selector/1 -> Complimentary Filter/2(theDot_gyro), Bus Creator/4  "<p>"
  Bus Selector/3 -> Complimentary Filter/3(psiDot_gyro), Bus Creator/6  "<r>"
  Bus Selector/2 -> Complimentary Filter/1(phiDot_gyro), Bus Creator/5  "<q>"
  Complimentary Filter/1(phi_est) -> Bus Creator/1  "roll"
  Complimentary Filter/2(theta_est) -> Bus Creator/2  "pitch"
  Complimentary Filter/3(psi_est) -> Bus Creator/3  "yaw"
  Subsystem1/2(phi_acc) -> Complimentary Filter/5(phiDot_acc)  "phi_acc"
  Subsystem1/1(theta_acc) -> Complimentary Filter/4(the_acc)  "theta_acc"
  Bus Selector/4 -> Subsystem1/1(x_acc)  "<x_acc>"
  Bus Selector/5 -> Subsystem1/2(y_acc)  "<y_acc>"
  Bus Selector/6 -> Subsystem1/3(z_acc)  "<z_acc>"
  Bus Creator/1 -> State Estimations/1

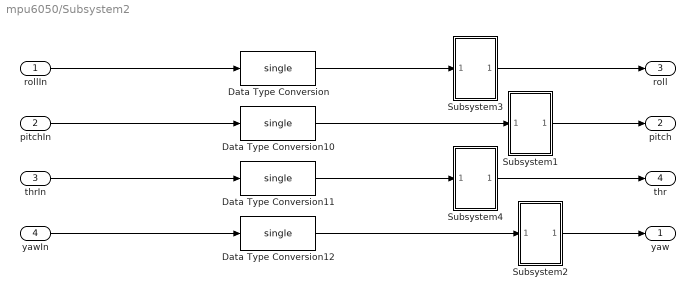
== system mpu6050/Subsystem2 ==
  rollIn : Inport
  pitchIn : Inport  Port=2
  thrIn : Inport  Port=3
  yawIn : Inport  Port=4
  Data Type Conversion{,10..12} (4 alike) : DataTypeConversion  OutDataTypeStr=single
  Subsystem1 : Subsystem
  Subsystem2 : Subsystem
  Subsystem3 : Subsystem
  Subsystem4 : Subsystem
  yaw : Outport
  pitch : Outport  Port=2
  roll : Outport  Port=3
  thr : Outport  Port=4
  wires:
  Subsystem1/1(Out1) -> pitch/1
  Subsystem3/1(Out1) -> roll/1
  pitchIn/1 -> Data Type Conversion10/1
  yawIn/1 -> Data Type Conversion12/1
  rollIn/1 -> Data Type Conversion/1
  Data Type Conversion11/1 -> Subsystem4/1(In1)
  Data Type Conversion/1 -> Subsystem3/1(In1)
  Data Type Conversion12/1 -> Subsystem2/1(In1)
  Data Type Conversion10/1 -> Subsystem1/1(In1)
  thrIn/1 -> Data Type Conversion11/1
  Subsystem4/1(Out1) -> thr/1
  Subsystem2/1(Out1) -> yaw/1

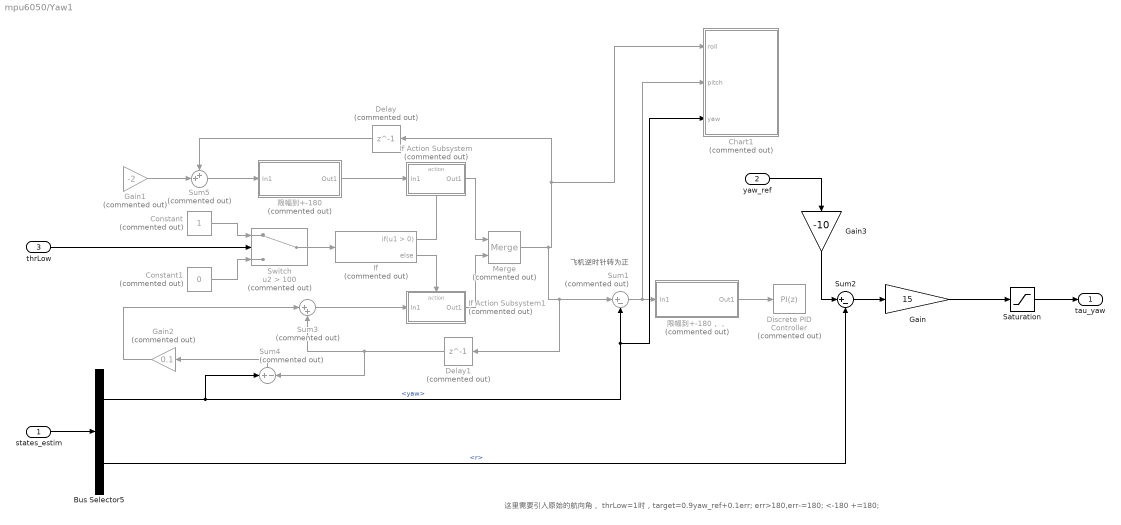
== system mpu6050/Yaw1 ==
  note: 飞机逆时针转为正
  note: 这里需要引入原始的航向角，
      | thrLow=1时，target=0.9yaw_ref+0.1err;
      | err>180,err-=180;
      | <-180 +=180;
  states_estim : Inport
  yaw_ref : Inport  Port=2
  thrLow : Inport  Port=3
  Bus Selector5 : BusSelector  OutputSignals=yaw,r
  Chart1 : Stateflow chart  Commented=on  TreatAsAtomicUnit=on
  Constant : Constant  Commented=on  OutDataTypeStr=int8
  Constant1 : Constant  Commented=on  Value=0  OutDataTypeStr=int8
  Delay : Delay  Commented=on  DelayLength=1
  Delay1 : Delay  Commented=on  DelayLength=1
  Discrete PID Controller : simulink/Continuous/PID Controller  Commented=on  Controller=PI  TimeDomain=Discrete-time  SampleTime=-1  IntegratorMethod=Forward Euler  FilterMethod=Forward Euler  Form=Parallel  UseFilter=on  ControllerParametersSource=internal  P=0.8  I=0  D=0  N=100  InitialConditionSource=internal  InitialConditionForIntegrator=0  InitialConditionForFilter=0  ExternalReset=none  LimitOutput=off  UpperSaturationLimit=inf  LowerSaturationLimit=-inf  LinearizeAsGain=off  AntiWindupMode=none  Kb=1  TrackingMode=off  Kt=1  PParamMin=[]  PParamMax=[]  IParamMin=[]  IParamMax=[]  DParamMin=[]  DParamMax=[]  NParamMin=[]  NParamMax=[]  KbParamMin=[]  KbParamMax=[]  KtParamMin=[]  KtParamMax=[]  POutMin=[]  POutMax=[]  IOutMin=[]  IOutMax=[]  DOutMin=[]  DOutMax=[]  NOutMin=[]  NOutMax=[]  KbOutMin=[]  KbOutMax=[]  KtOutMin=[]  KtOutMax=[]  IntegratorOutMin=[]  IntegratorOutMax=[]  FilterOutMin=[]  FilterOutMax=[]  SumOutMin=[]  SumOutMax=[]  SumI1OutMin=[]  SumI1OutMax=[]  SumI2OutMin=[]  SumI2OutMax=[]  SumI3OutMin=[]  SumI3OutMax=[]  SumDOutMin=[]  SumDOutMax=[]  SaturationOutMin=[]  SaturationOutMax=[]  IntegratorContinuousStateAttributes=''  IntegratorStateMustResolveToSignalObject=off  IntegratorRTWStateStorageClass=Auto  FilterContinuousStateAttributes=''  FilterStateMustResolveToSignalObject=off  FilterRTWStateStorageClass=Auto  DifferentiatorICPrevScaledInput=0  DifferentiatorOutMin=[]  DifferentiatorOutMax=[]  InitialConditionSetting=State (most efficient)  FilterDiffOutCoefMin=[]  FilterDiffOutCoefMax=[]  SumDenOutMin=[]  SumDenOutMax=[]  SumNumOutMin=[]  SumNumOutMax=[]  ReciprocalOutMin=[]  ReciprocalOutMax=[]  DivideOutMin=[]  DivideOutMax=[]  TunerSelectOption=Transfer Function Based (PID Tuner App)
  Gain : Gain  Gain=15
  Gain1 : Gain  Commented=on  Gain=-2
  Gain2 : Gain  Commented=on  Gain=0.1
  Gain3 : Gain  Gain=-10
  If : If  Commented=on
  If Action Subsystem : Subsystem  Commented=on  TreatAsAtomicUnit=on
  If Action Subsystem1 : Subsystem  Commented=on  TreatAsAtomicUnit=on
  Merge : Merge  Commented=on
  Saturation : Saturate  UpperLimit=300  LowerLimit=-300
  Sum1 : Sum  Commented=on  Inputs=|+-
  Sum2 : Sum  Inputs=|+-
  Sum3 : Sum  Commented=on  Inputs=|++
  Sum4 : Sum  Commented=on  Inputs=+|-
  Sum5 : Sum  Commented=on  Inputs=++|
  Switch : Switch  Commented=on  Criteria=u2 > Threshold  Threshold=100
  限幅到+-180 : Subsystem  Commented=on
  限幅到+-180，， : Subsystem  Commented=on
  tau_yaw : Outport
  wires:
  Gain/1 -> Saturation/1
  Sum2/1 -> Gain/1
  states_estim/1 -> Bus Selector5/1
  Bus Selector5/2 -> Sum2/2  "<r>"
  thrLow/1 -> Switch/2
  Constant/1 -> Switch/1
  Constant1/1 -> Switch/3
  Saturation/1 -> tau_yaw/1
  Switch/1 -> If/1
  If/1 -> If Action Subsystem/Action
  If Action Subsystem/1(Out1) -> Merge/1
  If/2 -> If Action Subsystem1/Action
  If Action Subsystem1/1(Out1) -> Merge/2
  Sum1/1 -> Chart1/2(pitch), 限幅到+-180，，/1(In1)
  Bus Selector5/1 -> Chart1/3(yaw), Sum1/2, Sum4/1  "<yaw>"
  Sum3/1 -> If Action Subsystem1/1(In1)
  限幅到+-180/1(Out1) -> If Action Subsystem/1(In1)
  限幅到+-180，，/1(Out1) -> Discrete PID Controller/1
  Sum5/1 -> 限幅到+-180/1(In1)
  ? -> Gain1/1
  Delay/1 -> Sum5/1
  Delay1/1 -> Sum3/2, Sum4/2
  Sum4/1 -> Gain2/1
  Gain2/1 -> Sum3/1
  Merge/1 -> Delay1/1, Sum1/1, Chart1/1(roll), Delay/1
  Gain1/1 -> Sum5/2
  yaw_ref/1 -> Gain3/1
  Gain3/1 -> Sum2/1

== system mpu6050/data scaling1 ==
  note: For simulation, no
      | offset value is calculated.
  In1 : Inport
  Bus Creator : BusCreator  Inputs=6
  Bus Selector : BusSelector  OutputSignals=gx_filt,gy_filt,gz_filt,ax_filt,ay_filt,az_filt
  Demux : Demux  Outputs=3
  Demux1 : Demux  Outputs=3
  Gain : Gain  Gain=pi/(180*16.4)
  Gain1 : Gain  Gain=9.81/16384
  Mux1 : Mux  Inputs=3
  Mux2 : Mux  Inputs=3
  Out1 : Outport
  wires:
  In1/1 -> Bus Selector/1
  Bus Selector/1 -> Mux1/1  "<gx_filt>"
  Bus Selector/2 -> Mux1/2  "<gy_filt>"
  Bus Selector/3 -> Mux1/3  "<gz_filt>"
  Bus Selector/4 -> Mux2/1  "<ax_filt>"
  Bus Selector/5 -> Mux2/2  "<ay_filt>"
  Bus Selector/6 -> Mux2/3  "<az_filt>"
  Mux2/1 -> Gain1/1
  Mux1/1 -> Gain/1
  Gain1/1 -> Demux1/1
  Gain/1 -> Demux/1
  Demux/1 -> Bus Creator/1  "p"
  Demux/2 -> Bus Creator/2  "q"
  Demux/3 -> Bus Creator/3  "r"
  Demux1/1 -> Bus Creator/4  "x_acc"
  Demux1/2 -> Bus Creator/5  "y_acc"
  Demux1/3 -> Bus Creator/6  "z_acc"
  Bus Creator/1 -> Out1/1

== system mpu6050/judgeLock2 ==
  In1 : Inport
  Constant3 : Constant  OutDataTypeStr=int8
  Constant4 : Constant  Value=0  OutDataTypeStr=int8
  GPIO_Write : GPIO_Lib/GPIO_Write  Port_name=GPIOA  Pin0=off  Toggle_Pin0=off  Pin1=off  Toggle_Pin1=off  Pin2=off  Toggle_Pin2=off  Pin3=off  Toggle_Pin3=off  Pin4=off  Toggle_Pin4=off  Pin5=off  Toggle_Pin5=off  Pin6=off  Toggle_Pin6=off  Pin7=off  Toggle_Pin7=off  Pin8=on  Toggle_Pin8=off  Pin9=off  Toggle_Pin9=off  Pin10=off  Toggle_Pin10=off  Pin11=on  Toggle_Pin11=off  Pin12=off  Toggle_Pin12=off  Pin13=off  Toggle_Pin13=off  Pin14=off  Toggle_Pin14=off  Pin15=off  Toggle_Pin15=off  PinList="GPIOA4   8  11  12GPIOB1  2  3  6  7"
      settings: SourceProductName=Target Support Package - STM32 Adapter
  GPIO_Write1 : GPIO_Lib/GPIO_Write  Port_name=GPIOB  Pin0=off  Toggle_Pin0=off  Pin1=on  Toggle_Pin1=off  Pin2=off  Toggle_Pin2=off  Pin3=on  Toggle_Pin3=off  Pin4=off  Toggle_Pin4=off  Pin5=off  Toggle_Pin5=off  Pin6=off  Toggle_Pin6=off  Pin7=off  Toggle_Pin7=off  Pin8=off  Toggle_Pin8=off  Pin9=off  Toggle_Pin9=off  Pin10=off  Toggle_Pin10=off  Pin11=off  Toggle_Pin11=off  Pin12=off  Toggle_Pin12=off  Pin13=off  Toggle_Pin13=off  Pin14=off  Toggle_Pin14=off  Pin15=off  Toggle_Pin15=off  PinList="GPIOA4   8  11  12GPIOB1  2  3  6  7"
      settings: SourceProductName=Target Support Package - STM32 Adapter
  If : If
  If Action Subsystem : Subsystem  TreatAsAtomicUnit=on
  If Action Subsystem1 : Subsystem  TreatAsAtomicUnit=on
  Merge : Merge
  wires:
  In1/1 -> If/1
  Constant4/1 -> If Action Subsystem1/1(In1)
  Constant3/1 -> If Action Subsystem/1(In1)
  If Action Subsystem1/1(Out1) -> Merge/2
  If/1 -> If Action Subsystem/Action
  If/2 -> If Action Subsystem1/Action
  If Action Subsystem/1(Out1) -> Merge/1
  Merge/1 -> GPIO_Write/1, GPIO_Write/2, GPIO_Write1/2, GPIO_Write1/1

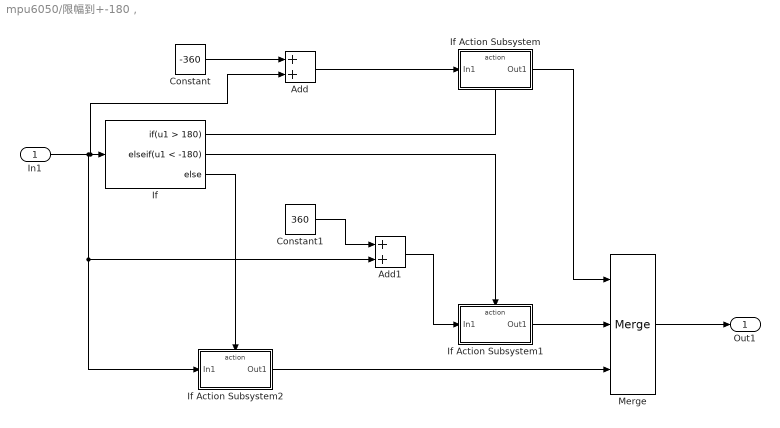
== system mpu6050/限幅到+-180， ==
  In1 : Inport  OutDataTypeStr=single
  Add : Sum
  Add1 : Sum
  Constant : Constant  Value=-360  OutDataTypeStr=single
  Constant1 : Constant  Value=360  OutDataTypeStr=single
  If : If  IfExpression=u1 > 180  ElseIfExpressions=u1 < -180
  If Action Subsystem : Subsystem  TreatAsAtomicUnit=on
  If Action Subsystem1 : Subsystem  TreatAsAtomicUnit=on
  If Action Subsystem2 : Subsystem  TreatAsAtomicUnit=on
  Merge : Merge  Inputs=3
  Out1 : Outport
  wires:
  Merge/1 -> Out1/1
  Add1/1 -> If Action Subsystem1/1(In1)
  If Action Subsystem2/1(Out1) -> Merge/3
  Constant1/1 -> Add1/1
  If Action Subsystem1/1(Out1) -> Merge/2
  Add/1 -> If Action Subsystem/1(In1)
  Constant/1 -> Add/1
  If Action Subsystem/1(Out1) -> Merge/1
  If/3 -> If Action Subsystem2/Action
  If/2 -> If Action Subsystem1/Action
  If/1 -> If Action Subsystem/Action
  In1/1 -> If/1, Add/2, If Action Subsystem2/1(In1), Add1/2

== system mpu6050/Attitude1/Low Pass Filter1 ==
  GyroMeasure : Inport
  Demux : Demux  Outputs=2
  Digital Low Pass Filter1 : DiscreteTransferFcn  Numerator=[0.04877]  Denominator=[1 -0.9512]  OutDataTypeStr=int16
  Digital Low Pass Filter2 : DiscreteTransferFcn  Numerator=[0.04877]  Denominator=[1 -0.9512]  OutDataTypeStr=int16
  Mux3 : Mux  Inputs=2
  GyroFiltered : Outport
  wires:
  Mux3/1 -> GyroFiltered/1
  Demux/1 -> Digital Low Pass Filter2/1
  GyroMeasure/1 -> Demux/1
  Demux/2 -> Digital Low Pass Filter1/1
  Digital Low Pass Filter2/1 -> Mux3/1
  Digital Low Pass Filter1/1 -> Mux3/2

== system mpu6050/PWM1/Subsystem ==
  In1 : Inport
  Demux : Demux
  Divide : Product  Inputs=*/
  Gain : Gain  Gain=1000
  If : If  IfExpression=u1 > 1000
  If Action Subsystem : Subsystem  TreatAsAtomicUnit=on
  If Action Subsystem1 : Subsystem  TreatAsAtomicUnit=on
  Merge : Merge
  Min : MinMax  Function=max  Inputs=4
  Out1 : Outport
  wires:
  Demux/4 -> Min/4
  In1/1 -> Divide/1, If Action Subsystem1/1(In1), Demux/1
  Demux/1 -> Min/1
  Demux/2 -> Min/2
  Demux/3 -> Min/3
  If/1 -> If Action Subsystem/Action
  If/2 -> If Action Subsystem1/Action
  If Action Subsystem/1(Out1) -> Merge/1
  If Action Subsystem1/1(Out1) -> Merge/2
  Min/1 -> Divide/2, If/1
  Gain/1 -> If Action Subsystem/1(In1)
  Divide/1 -> Gain/1
  Merge/1 -> Out1/1

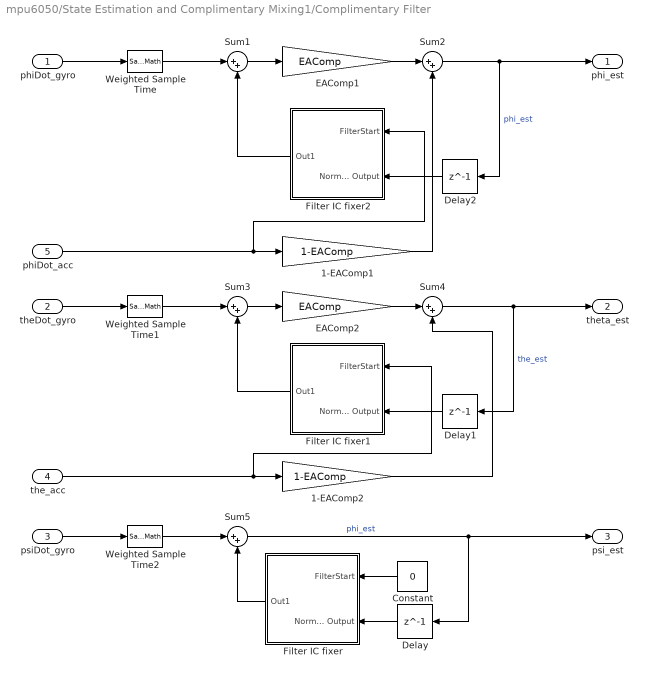
== system mpu6050/State Estimation and Complimentary Mixing1/Complimentary Filter ==
  phiDot_gyro : Inport
  theDot_gyro : Inport  Port=2
  psiDot_gyro : Inport  Port=3
  the_acc : Inport  Port=4
  phiDot_acc : Inport  Port=5
  1-EAComp1 : Gain  Gain=1-EAComp
  1-EAComp2 : Gain  Gain=1-EAComp
  Constant : Constant  Value=0  OutDataTypeStr=single
  Delay : Delay  DelayLength=1  InitialCondition=0
  Delay1 : Delay  DelayLength=1  InitialCondition=0
  Delay2 : Delay  DelayLength=1  InitialCondition=0
  EAComp1 : Gain  Gain=EAComp
  EAComp2 : Gain  Gain=EAComp
  Filter IC fixer : Subsystem
  Filter IC fixer1 : Subsystem
  Filter IC fixer2 : Subsystem
  Sum{1..4} (4 alike) : Sum  Inputs=|++
  Sum5 : Sum  Inputs=|++  OutDataTypeStr=single
  Weighted Sample Time : SampleTimeMath  TsampMathOp=*
  Weighted Sample Time1 : SampleTimeMath  TsampMathOp=*
  Weighted Sample Time2 : SampleTimeMath  TsampMathOp=*
  phi_est : Outport
  theta_est : Outport  Port=2
  psi_est : Outport  Port=3  OutDataTypeStr=single
  wires:
  Weighted Sample Time/1 -> Sum1/1
  Sum1/1 -> EAComp1/1
  Sum2/1 -> Delay2/1, phi_est/1  "phi_est"
  1-EAComp1/1 -> Sum2/2
  phiDot_gyro/1 -> Weighted Sample Time/1
  phiDot_acc/1 -> Filter IC fixer2/1(FilterStart), 1-EAComp1/1
  EAComp1/1 -> Sum2/1
  Weighted Sample Time1/1 -> Sum3/1
  Sum3/1 -> EAComp2/1
  Sum4/1 -> Delay1/1, theta_est/1  "the_est"
  1-EAComp2/1 -> Sum4/2
  theDot_gyro/1 -> Weighted Sample Time1/1
  the_acc/1 -> 1-EAComp2/1, Filter IC fixer1/1(FilterStart)
  EAComp2/1 -> Sum4/1
  psiDot_gyro/1 -> Weighted Sample Time2/1
  Weighted Sample Time2/1 -> Sum5/1
  Sum5/1 -> Delay/1, psi_est/1  "phi_est"
  Delay/1 -> Filter IC fixer/2(Normal Output)
  Filter IC fixer/1(Out1) -> Sum5/2
  Constant/1 -> Filter IC fixer/1(FilterStart)
  Filter IC fixer1/1(Out1) -> Sum3/2
  Filter IC fixer2/1(Out1) -> Sum1/2
  Delay1/1 -> Filter IC fixer1/2(Normal Output)
  Delay2/1 -> Filter IC fixer2/2(Normal Output)

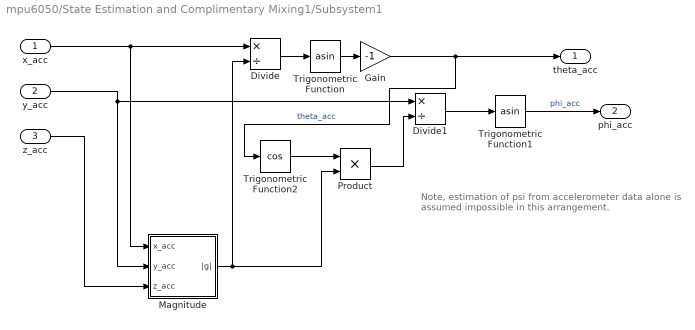
== system mpu6050/State Estimation and Complimentary Mixing1/Subsystem1 ==
  note: Note, estimation of psi from accelerometer data alone
      | is assumed impossible in this arrangement.
  x_acc : Inport
  y_acc : Inport  Port=2
  z_acc : Inport  Port=3
  Divide : Product  Inputs=*/
  Divide1 : Product  Inputs=*/
  Gain : Gain  Gain=-1
  Magnitude : Subsystem
  Product : Product
  Trigonometric Function : Trigonometry  Operator=asin  OutputSignalType=real
  Trigonometric Function1 : Trigonometry  Operator=asin  OutputSignalType=real
  Trigonometric Function2 : Trigonometry  Operator=cos  OutputSignalType=real
  theta_acc : Outport
  phi_acc : Outport  Port=2
  wires:
  Divide/1 -> Trigonometric Function/1
  Magnitude/1(|g|) -> Product/2, Divide/2
  Trigonometric Function2/1 -> Product/1
  Trigonometric Function/1 -> Gain/1
  y_acc/1 -> Magnitude/2(y_acc), Divide1/1
  z_acc/1 -> Magnitude/3(z_acc)
  Divide1/1 -> Trigonometric Function1/1
  Product/1 -> Divide1/2
  Trigonometric Function1/1 -> phi_acc/1  "phi_acc"
  x_acc/1 -> Magnitude/1(x_acc), Divide/1
  Gain/1 -> theta_acc/1, Trigonometric Function2/1  "theta_acc"

== system mpu6050/Subsystem2/Subsystem1 ==
  In1 : Inport
  Constant3 : Constant  Value=1500  OutDataTypeStr=single
  Constant4 : Constant  Value=500  OutDataTypeStr=single
  Dead Zone : DeadZone  LowerValue=-70  UpperValue=70  SaturateOnIntegerOverflow=on
  Divide1 : Product  Inputs=*/
  Saturation4 : Saturate  UpperLimit=2000  LowerLimit=1000
  Sum1 : Sum  Inputs=|+-
  Out1 : Outport
  wires:
  Divide1/1 -> Out1/1
  Dead Zone/1 -> Divide1/1
  Constant3/1 -> Sum1/2
  Saturation4/1 -> Sum1/1
  Constant4/1 -> Divide1/2
  In1/1 -> Saturation4/1
  Sum1/1 -> Dead Zone/1
